simulink library "nmc"  (R2015b)
settings: Solver=ode45  SolverMode=SingleTasking  StartTime=0.0  StopTime=10.0  RelTol=1e-3
undefined symbols (not defined in the file): AFOFS_DIM, alphaFmGas, alphaFmGlu, alphaFmHam, alphaFmSol, alphaFmVas, alphaLceHam, alphaLceHfl, alphaLceTa, alphaLceTa1, Amp, amp_var, c, c_jointstop, CPG, D1G_HAT, DeltaThRef, eref, FmaxGAS, FmaxGLU, FmaxHAM, FmaxHFL, FmaxSOL, FmaxTA, FmaxVAS, freq, freq_var, GainDeltaTheta, GainGAS, GainGLU, GainHAM, GainHAMHFL, GainHFL, GainKneOverExt, GainSOL, GainSOLTA, GainTA, GainVAS, K, K_swing, KneePh23Offset, LceOffsetHAM, LceOffsetHFL, LceOffsetTA, left, LongDelay, loptGAS, loptGLU, loptHAM, loptHFL, loptSOL, loptTA, loptVAS, Lphi230, lslackGAS, lslackGLU, lslackHAM, lslackHFL, lslackSOL, lslackTA ... (+66)
libraries: nmc x94, simulink x29, simulink_extras x17
(part 2 of 5)

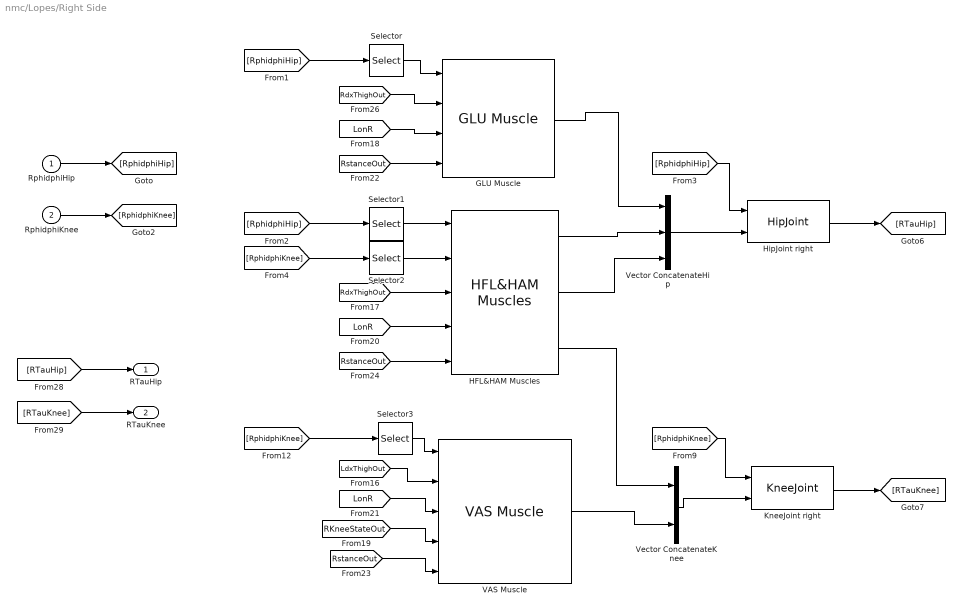
== system nmc/Lopes/Right Side ==
  RphidphiHip : Inport
  RphidphiKnee : Inport  Port=2
  GLU Muscle : nmc/NMC Muscles/GLU Muscle  StimGluSide=StimGLUR  GotoTag=GLUR_VM
  HFL&HAM Muscles : nmc/NMC Muscles/HFL&HAM Muscles  StimHAMSide=StimHAMR  StimHFLSide=StimHFLR  HAMVM=HAMR_VM  HFLVM=HFLR_VM
  HipJoint right : nmc/NMC Joints/HipJoint
  KneeJoint right : nmc/NMC Joints/KneeJoint
  Selector{,1..3} (4 alike) : Selector  InputPortWidth=2  IndexOptions=Index vector (dialog)  Indices=[1 ]  OutputSizes=1
  VAS Muscle : nmc/NMC Muscles/VAS Muscle  VariableName=StimVASR  VASVM=VASR_VM
  Vector ConcatenateHip : Concatenate  NumInputs=3
  Vector ConcatenateKnee : Concatenate
  RTauHip : Outport
  RTauKnee : Outport  Port=2
  wires:
  Vector ConcatenateHip/1 -> HipJoint right/2
  [RphidphiKnee] -> KneeJoint right/1
  Selector1/1 -> HFL&HAM Muscles/1
  [LdxThighOut] -> VAS Muscle/2
  Vector ConcatenateKnee/1 -> KneeJoint right/2
  Selector3/1 -> VAS Muscle/1
  VAS Muscle/1 -> Vector ConcatenateKnee/2
  HFL&HAM Muscles/1 -> Vector ConcatenateHip/2
  GLU Muscle/1 -> Vector ConcatenateHip/1
  [LonR] -> VAS Muscle/3
  [RphidphiKnee] -> Selector3/1
  [RKneeStateOut] -> VAS Muscle/4
  HFL&HAM Muscles/3 -> Vector ConcatenateKnee/1
  Selector/1 -> GLU Muscle/1
  HFL&HAM Muscles/2 -> Vector ConcatenateHip/3
  Selector2/1 -> HFL&HAM Muscles/2
  [RphidphiHip] -> Selector1/1
  [RstanceOut] -> VAS Muscle/5
  [RphidphiHip] -> Selector/1
  [RphidphiHip] -> HipJoint right/1
  [RphidphiKnee] -> Selector2/1
  HipJoint right/1 -> [RTauHip]
  KneeJoint right/1 -> [RTauKnee]
  [RdxThighOut] -> GLU Muscle/2
  [LonR] -> GLU Muscle/3
  [RstanceOut] -> GLU Muscle/4
  [RdxThighOut] -> HFL&HAM Muscles/3
  [LonR] -> HFL&HAM Muscles/4
  [RstanceOut] -> HFL&HAM Muscles/5
  RphidphiHip/1 -> [RphidphiHip]
  RphidphiKnee/1 -> [RphidphiKnee]
  [RTauHip] -> RTauHip/1
  [RTauKnee] -> RTauKnee/1

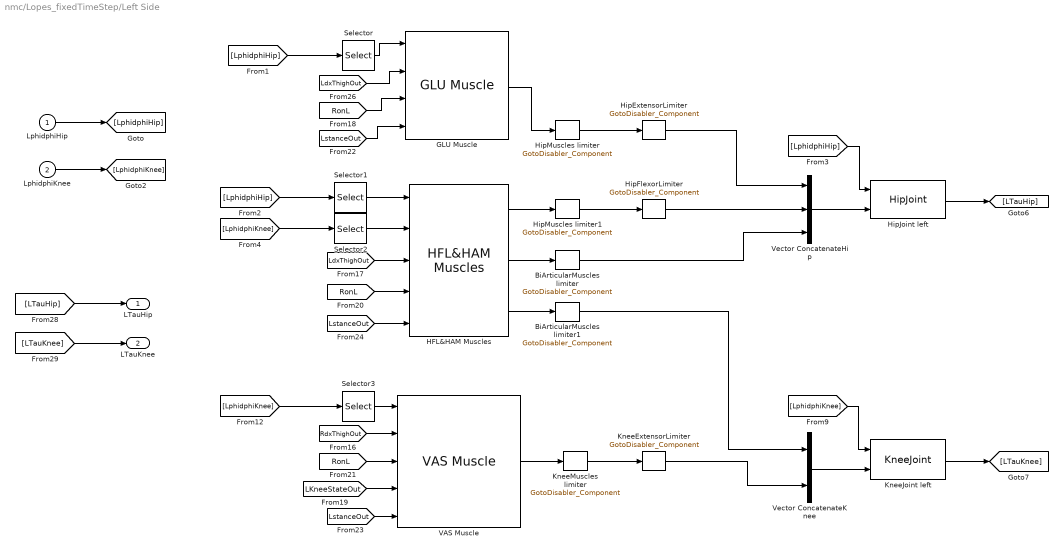
== system nmc/Lopes_fixedTimeStep/Left Side ==
  LphidphiHip : Inport
  LphidphiKnee : Inport  Port=2
  BiArticularMuscles limiter : nmc/GotoDisabler_Component  GotoTag=NMC_BiArticularMuscles_Percentage
  BiArticularMuscles limiter1 : nmc/GotoDisabler_Component  GotoTag=NMC_BiArticularMuscles_Percentage
  GLU Muscle : nmc/NMC Muscles/GLU Muscle  StimGluSide=StimGLUL  GotoTag=GLUR_VM
  HFL&HAM Muscles : nmc/NMC Muscles/HFL&HAM Muscles  StimHAMSide=StimHAML  StimHFLSide=StimHFLL  HAMVM=HAMR_VM  HFLVM=HFLR_VM
  HipExtensorLimiter : nmc/GotoDisabler_Component  GotoTag=NMC_HipExtensors_Percentage
  HipFlexorLimiter : nmc/GotoDisabler_Component  GotoTag=NMC_HipFlexors_Percentage
  HipJoint left : nmc/NMC Joints/HipJoint
  HipMuscles limiter : nmc/GotoDisabler_Component  GotoTag=NMC_HipMuscles_Percentage
  HipMuscles limiter1 : nmc/GotoDisabler_Component  GotoTag=NMC_HipMuscles_Percentage
  KneeExtensorLimiter : nmc/GotoDisabler_Component  GotoTag=NMC_KneeExtensors_Percentage
  KneeJoint left : nmc/NMC Joints/KneeJoint
  KneeMuscles limiter : nmc/GotoDisabler_Component  GotoTag=NMC_KneeMuscles_Percentage
  Selector{,1..3} (4 alike) : Selector  InputPortWidth=2  IndexOptions=Index vector (dialog)  Indices=[1 ]  OutputSizes=1
  VAS Muscle : nmc/NMC Muscles/VAS Muscle  VariableName=StimVASL  VASVM=VASR_VM
  Vector ConcatenateHip : Concatenate  NumInputs=3
  Vector ConcatenateKnee : Concatenate
  LTauHip : Outport
  LTauKnee : Outport  Port=2
  wires:
  KneeExtensorLimiter/1 -> Vector ConcatenateKnee/2
  BiArticularMuscles limiter1/1 -> Vector ConcatenateKnee/1
  HipFlexorLimiter/1 -> Vector ConcatenateHip/2
  HipExtensorLimiter/1 -> Vector ConcatenateHip/1
  KneeMuscles limiter/1 -> KneeExtensorLimiter/1
  BiArticularMuscles limiter/1 -> Vector ConcatenateHip/3
  HipMuscles limiter1/1 -> HipFlexorLimiter/1
  HipMuscles limiter/1 -> HipExtensorLimiter/1
  HFL&HAM Muscles/3 -> BiArticularMuscles limiter1/1
  GLU Muscle/1 -> HipMuscles limiter/1
  [LTauKnee] -> LTauKnee/1
  [LTauHip] -> LTauHip/1
  LphidphiKnee/1 -> [LphidphiKnee]
  LphidphiHip/1 -> [LphidphiHip]
  [LdxThighOut] -> HFL&HAM Muscles/3
  [RonL] -> GLU Muscle/3
  [LstanceOut] -> GLU Muscle/4
  [LdxThighOut] -> GLU Muscle/2
  KneeJoint left/1 -> [LTauKnee]
  HipJoint left/1 -> [LTauHip]
  [LphidphiKnee] -> Selector2/1
  [LphidphiHip] -> HipJoint left/1
  [LphidphiHip] -> Selector/1
  [LstanceOut] -> VAS Muscle/5
  [LphidphiHip] -> Selector1/1
  Selector2/1 -> HFL&HAM Muscles/2
  HFL&HAM Muscles/2 -> BiArticularMuscles limiter/1
  Selector/1 -> GLU Muscle/1
  [LKneeStateOut] -> VAS Muscle/4
  [RonL] -> HFL&HAM Muscles/4
  [LphidphiKnee] -> Selector3/1
  [RonL] -> VAS Muscle/3
  [LstanceOut] -> HFL&HAM Muscles/5
  HFL&HAM Muscles/1 -> HipMuscles limiter1/1
  VAS Muscle/1 -> KneeMuscles limiter/1
  Selector3/1 -> VAS Muscle/1
  Vector ConcatenateKnee/1 -> KneeJoint left/2
  [RdxThighOut] -> VAS Muscle/2
  Selector1/1 -> HFL&HAM Muscles/1
  [LphidphiKnee] -> KneeJoint left/1
  Vector ConcatenateHip/1 -> HipJoint left/2

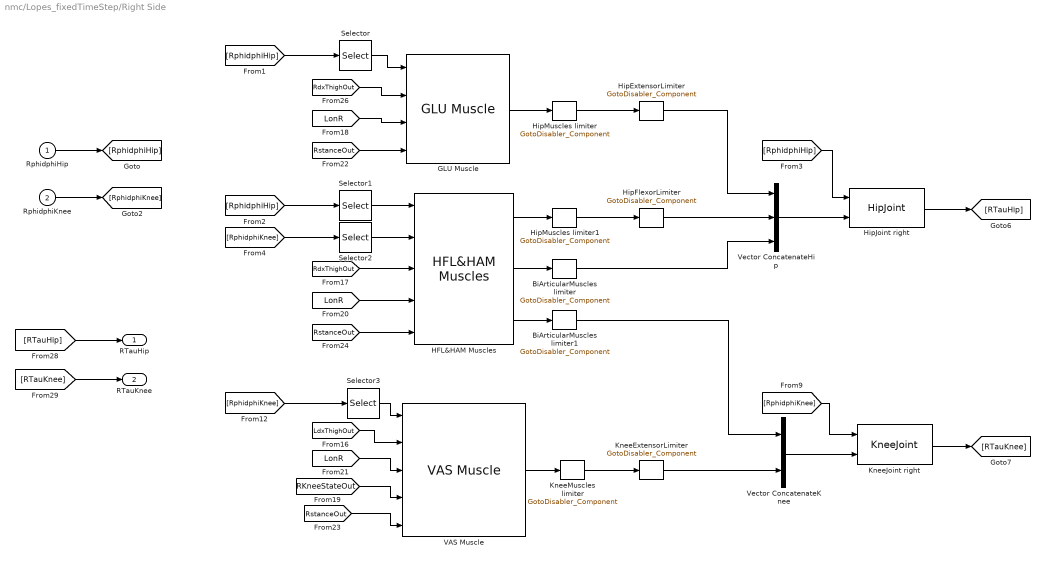
== system nmc/Lopes_fixedTimeStep/Right Side ==
  RphidphiHip : Inport
  RphidphiKnee : Inport  Port=2
  BiArticularMuscles limiter : nmc/GotoDisabler_Component  GotoTag=NMC_BiArticularMuscles_Percentage
  BiArticularMuscles limiter1 : nmc/GotoDisabler_Component  GotoTag=NMC_BiArticularMuscles_Percentage
  GLU Muscle : nmc/NMC Muscles/GLU Muscle  StimGluSide=StimGLUR  GotoTag=GLUR_VM
  HFL&HAM Muscles : nmc/NMC Muscles/HFL&HAM Muscles  StimHAMSide=StimHAMR  StimHFLSide=StimHFLR  HAMVM=HAMR_VM  HFLVM=HFLR_VM
  HipExtensorLimiter : nmc/GotoDisabler_Component  GotoTag=NMC_HipExtensors_Percentage
  HipFlexorLimiter : nmc/GotoDisabler_Component  GotoTag=NMC_HipFlexors_Percentage
  HipJoint right : nmc/NMC Joints/HipJoint
  HipMuscles limiter : nmc/GotoDisabler_Component  GotoTag=NMC_HipMuscles_Percentage
  HipMuscles limiter1 : nmc/GotoDisabler_Component  GotoTag=NMC_HipMuscles_Percentage
  KneeExtensorLimiter : nmc/GotoDisabler_Component  GotoTag=NMC_KneeExtensors_Percentage
  KneeJoint right : nmc/NMC Joints/KneeJoint
  KneeMuscles limiter : nmc/GotoDisabler_Component  GotoTag=NMC_KneeMuscles_Percentage
  Selector{,1..3} (4 alike) : Selector  InputPortWidth=2  IndexOptions=Index vector (dialog)  Indices=[1 ]  OutputSizes=1
  VAS Muscle : nmc/NMC Muscles/VAS Muscle  VariableName=StimVASR  VASVM=VASR_VM
  Vector ConcatenateHip : Concatenate  NumInputs=3
  Vector ConcatenateKnee : Concatenate
  RTauHip : Outport
  RTauKnee : Outport  Port=2
  wires:
  KneeExtensorLimiter/1 -> Vector ConcatenateKnee/2
  BiArticularMuscles limiter1/1 -> Vector ConcatenateKnee/1
  HipFlexorLimiter/1 -> Vector ConcatenateHip/2
  HipExtensorLimiter/1 -> Vector ConcatenateHip/1
  KneeMuscles limiter/1 -> KneeExtensorLimiter/1
  BiArticularMuscles limiter/1 -> Vector ConcatenateHip/3
  HipMuscles limiter1/1 -> HipFlexorLimiter/1
  HipMuscles limiter/1 -> HipExtensorLimiter/1
  [RTauKnee] -> RTauKnee/1
  [RTauHip] -> RTauHip/1
  RphidphiKnee/1 -> [RphidphiKnee]
  RphidphiHip/1 -> [RphidphiHip]
  [RstanceOut] -> HFL&HAM Muscles/5
  [LonR] -> HFL&HAM Muscles/4
  [RdxThighOut] -> HFL&HAM Muscles/3
  [RstanceOut] -> GLU Muscle/4
  [LonR] -> GLU Muscle/3
  [RdxThighOut] -> GLU Muscle/2
  KneeJoint right/1 -> [RTauKnee]
  HipJoint right/1 -> [RTauHip]
  [RphidphiKnee] -> Selector2/1
  [RphidphiHip] -> HipJoint right/1
  [RphidphiHip] -> Selector/1
  [RstanceOut] -> VAS Muscle/5
  [RphidphiHip] -> Selector1/1
  Selector2/1 -> HFL&HAM Muscles/2
  HFL&HAM Muscles/2 -> BiArticularMuscles limiter/1
  Selector/1 -> GLU Muscle/1
  HFL&HAM Muscles/3 -> BiArticularMuscles limiter1/1
  [RKneeStateOut] -> VAS Muscle/4
  [RphidphiKnee] -> Selector3/1
  [LonR] -> VAS Muscle/3
  GLU Muscle/1 -> HipMuscles limiter/1
  HFL&HAM Muscles/1 -> HipMuscles limiter1/1
  VAS Muscle/1 -> KneeMuscles limiter/1
  Selector3/1 -> VAS Muscle/1
  Vector ConcatenateKnee/1 -> KneeJoint right/2
  [LdxThighOut] -> VAS Muscle/2
  Selector1/1 -> HFL&HAM Muscles/1
  [RphidphiKnee] -> KneeJoint right/1
  Vector ConcatenateHip/1 -> HipJoint right/2

== system nmc/NMC Joints/AnkleJoint ==
  note: Ankle Joint
  phidphiAnkle : Inport
  PreTauAnkle : Inport  Port=2
  " Ankle Joint Limits" : Subsystem
  Demux : Demux  Outputs=2
  GotoDisabler_Component : nmc/GotoDisabler_Component  GotoTag=EnableNMC_JointLimits
  LOG_TauAnkleLigament : Concatenate  NumInputs=1
  Sum : Sum  Inputs=|++
  Sum of Elements : Sum  Inputs=+
  TauAnkle : Outport
  wires:
  Demux/1 -> " Ankle Joint Limits"/1(phi [rad])
  Demux/2 -> " Ankle Joint Limits"/2(dphi [rad/s])
  PreTauAnkle/1 -> Sum of Elements/1
  phidphiAnkle/1 -> Demux/1
  " Ankle Joint Limits"/1(M_stop [Nm]) -> LOG_TauAnkleLigament/1
  Sum/1 -> TauAnkle/1
  Sum of Elements/1 -> Sum/2
  LOG_TauAnkleLigament/1 -> GotoDisabler_Component/1
  GotoDisabler_Component/1 -> Sum/1

== system nmc/NMC Joints/HipJoint ==
  note: Hip Joint
  phidphiHip : Inport
  PreTauHip : Inport  Port=2
  Demux2 : Demux  Outputs=2
  GotoDisabler_Component : nmc/GotoDisabler_Component  GotoTag=DisableNMC_JointLimits
  Hip Joint Limits : Subsystem
  Sum of Elements : Sum  Inputs=+
  Sum16 : Sum  Inputs=|++
  TauHip : Outport
  wires:
  phidphiHip/1 -> Demux2/1
  Demux2/1 -> Hip Joint Limits/1(phi [rad])
  Demux2/2 -> Hip Joint Limits/2(dphi [rad/s])
  Hip Joint Limits/1(M_stop [Nm]) -> GotoDisabler_Component/1
  Sum16/1 -> TauHip/1
  PreTauHip/1 -> Sum of Elements/1
  Sum of Elements/1 -> Sum16/2
  GotoDisabler_Component/1 -> Sum16/1

== system nmc/NMC Joints/KneeJoint ==
  note: Knee Joint
  phidphiKnee : Inport
  PreTauKnee : Inport  Port=2
  Demux1 : Demux  Outputs=2
  Gain : Gain  Gain=-1
  GotoDisabler_Component : nmc/GotoDisabler_Component  GotoTag=DisableNMC_JointLimits
  Knee Joint Limits : Subsystem
  Sum : Sum  Inputs=|++
  Sum of Elements : Sum  Inputs=+
  TauKnee : Outport
  wires:
  Demux1/1 -> Knee Joint Limits/1(phi [rad])
  Demux1/2 -> Knee Joint Limits/2(dphi [rad/s])
  phidphiKnee/1 -> Demux1/1
  Knee Joint Limits/1(M_stop [Nm]) -> GotoDisabler_Component/1
  Sum/1 -> TauKnee/1
  PreTauKnee/1 -> Sum of Elements/1
  Sum of Elements/1 -> Gain/1
  Gain/1 -> Sum/2
  GotoDisabler_Component/1 -> Sum/1

== system nmc/NMC Muscles/GAS Muscle ==
  note: GAS Muscle
  phiKnee : Inport
  phiAnkle : Inport  Port=2
  StanceSwing : Inport  Port=3
  "GAS Actuation " : Subsystem
  GAS Control : Subsystem
  LOG_GasAnkle : Concatenate  NumInputs=1
  LOG_TauGasKnee : Concatenate  NumInputs=1
  StimGAS : ToWorkspace  VariableName=StimGAS  SaveFormat=Timeseries  SampleTime=-1
  TauGasKnee : Outport
  TauGasAnkle : Outport  Port=2
  wires:
  GAS Control/1(StimGAS) -> "GAS Actuation "/3(StimGas), StimGAS/1
  phiKnee/1 -> "GAS Actuation "/1(phiKnee)
  StanceSwing/1 -> GAS Control/2(StanceSwing)
  "GAS Actuation "/3(FmGas) -> GAS Control/1(FmGAS)
  "GAS Actuation "/2(TauGasAnkle) -> LOG_GasAnkle/1
  "GAS Actuation "/1(TauGasKnee) -> LOG_TauGasKnee/1
  phiAnkle/1 -> "GAS Actuation "/2(phiAnkle)
  LOG_TauGasKnee/1 -> TauGasKnee/1
  LOG_GasAnkle/1 -> TauGasAnkle/1

== system nmc/NMC Muscles/GLU Muscle ==
  note: GLU Muscle
  phiHip : Inport
  CLdxThigh : Inport  Port=2
  OLonCL : Inport  Port=3
  StanceSwing : Inport  Port=4
  GLU Actuation : Subsystem
  GLU Control : Subsystem
  LOG_TauGlu : Concatenate  NumInputs=1
  StimGLU : ToWorkspace  VariableName=StimGLUR  SaveFormat=Timeseries  SampleTime=-1
  TauGlu : Outport
  wires:
  GLU Actuation/1(TauGlu) -> LOG_TauGlu/1
  StanceSwing/1 -> GLU Control/6(StanceSwing)
  CLdxThigh/1 -> GLU Control/4(CLdxThigh)
  phiHip/1 -> GLU Actuation/1(phiHip)
  [dThetaDelayed] -> GLU Control/3(dTheta)
  [ThetaDelayed] -> GLU Control/2(Theta)
  OLonCL/1 -> GLU Control/5(OLonCL)
  GLU Actuation/2(FmGlu) -> GLU Control/1(FmGlu)
  GLU Control/1(StimGlu) -> StimGLU/1, GLU Actuation/2(StimGlu)
  LOG_TauGlu/1 -> TauGlu/1

== system nmc/NMC Muscles/HFL Muscle  ==
  note: HFL Muscle
  phiHip : Inport
  CLdxThigh : Inport  Port=2
  OLonCL : Inport  Port=3
  StanceSwing : Inport  Port=4
  HFL Actuation : Subsystem
  HFL Control : Subsystem
  LOG_TauHFL : Concatenate  NumInputs=1
  StimHFL : ToWorkspace  VariableName=StimHFL  SaveFormat=Timeseries  SampleTime=-1
  TauHFL : Outport
  wires:
  HFL Actuation/1(TauHFL) -> LOG_TauHFL/1
  phiHip/1 -> HFL Actuation/1(phiHip)
  StanceSwing/1 -> HFL Control/6(StanceSwing)
  OLonCL/1 -> HFL Control/5(OLonCL)
  CLdxThigh/1 -> HFL Control/4(CLdxThigh)
  [dThetaDelayed] -> HFL Control/3(dTheta)
  [ThetaDelayed] -> HFL Control/2(Theta)
  HFL Control/1(StimHFL) -> HFL Actuation/2(StimHFL), StimHFL/1
  HFL Actuation/2(LceHFL) -> HFL Control/1(LceHFL)
  LOG_TauHFL/1 -> TauHFL/1

== system nmc/NMC Muscles/HFL&HAM Muscles ==
  note: HFL&HAM Muscles
  phiHip : Inport
  phiKnee : Inport  Port=2
  CLdxThigh : Inport  Port=3
  OLonCL : Inport  Port=4
  StanceSwing : Inport  Port=5
  "HAM Actuation " : Subsystem
  HFL Actuation : Subsystem
  HFL&HAM Control : Subsystem
  LOG_TauHFL : Concatenate  NumInputs=1
  LOG_TauHamHip : Concatenate  NumInputs=1
  LOG_TauHamKnee : Concatenate  NumInputs=1
  StimHAM : ToWorkspace  VariableName=StimHAMR  SaveFormat=Timeseries  SampleTime=-1
  StimHFL : ToWorkspace  VariableName=StimHFLR  SaveFormat=Timeseries  SampleTime=-1
  TauHFL : Outport
  TauHamHip : Outport  Port=2
  TauHamKnee : Outport  Port=3
  wires:
  HFL&HAM Control/1(StimHFL) -> HFL Actuation/2(StimHFL), StimHFL/1
  "HAM Actuation "/3(LceHam) -> HFL&HAM Control/2(LceHam)
  "HAM Actuation "/4(FmHam) -> HFL&HAM Control/3(FmHam)
  HFL Actuation/2(LceHFL) -> HFL&HAM Control/1(LceHFL)
  OLonCL/1 -> HFL&HAM Control/7(OLonCL)
  "HAM Actuation "/1(TauHamHip) -> LOG_TauHamHip/1
  phiHip/1 -> HFL Actuation/1(phiHip), "HAM Actuation "/1(phiHip)
  "HAM Actuation "/2(TauHamKnee) -> LOG_TauHamKnee/1
  CLdxThigh/1 -> HFL&HAM Control/6(CLdxThigh)
  HFL Actuation/1(TauHFL) -> LOG_TauHFL/1
  phiKnee/1 -> "HAM Actuation "/2(phiKnee)
  [ThetaDelayed] -> HFL&HAM Control/4(Theta)
  [dThetaDelayed] -> HFL&HAM Control/5(dTheta)
  StanceSwing/1 -> HFL&HAM Control/8(StanceSwing)
  HFL&HAM Control/2(StimHAM) -> "HAM Actuation "/3(StimHam), StimHAM/1
  LOG_TauHFL/1 -> TauHFL/1
  LOG_TauHamHip/1 -> TauHamHip/1
  LOG_TauHamKnee/1 -> TauHamKnee/1

== system nmc/NMC Muscles/SOL&TA Muscles ==
  note: SOL&TA Muscles
  phiAnkle : Inport
  StanceSwing : Inport  Port=2
  LOG_StimSOL : Concatenate  NumInputs=1
  LOG_StimTA : Concatenate  NumInputs=1
  LOG_TauSOL : Concatenate  NumInputs=1
  LOG_TauTA : Concatenate  NumInputs=1
  SOL Actuation : Subsystem
  SOL&TA Control : Subsystem
  StimSOL : ToWorkspace  VariableName=StimSOL  SaveFormat=Timeseries  SampleTime=-1
  StimTA : ToWorkspace  VariableName=StimTA  SaveFormat=Timeseries  SampleTime=-1
  TA Actuation : Subsystem
  TauTA : Outport
  TauSOL : Outport  Port=2
  wires:
  SOL&TA Control/2(StimSOL) -> LOG_StimSOL/1
  SOL Actuation/2(FmSOL) -> SOL&TA Control/2(FmSOL)
  SOL Actuation/1(TauSOL) -> LOG_TauSOL/1
  SOL&TA Control/1(StimTA) -> LOG_StimTA/1
  StanceSwing/1 -> SOL&TA Control/3(StanceSwing)
  TA Actuation/1(LceTA) -> SOL&TA Control/1(LceTA)
  phiAnkle/1 -> TA Actuation/1(phiAnkle), SOL Actuation/1(phiAnkle)
  TA Actuation/2(TauTa) -> LOG_TauTA/1
  LOG_TauTA/1 -> TauTA/1
  LOG_TauSOL/1 -> TauSOL/1
  LOG_StimTA/1 -> StimTA/1, TA Actuation/2(StimTA)
  LOG_StimSOL/1 -> SOL Actuation/2(StimSOL), StimSOL/1

== system nmc/NMC Muscles/VAS Muscle ==
  note: VAS Muscle
  phiKnee : Inport
  OLdxThigh : Inport  Port=2
  OLonCL : Inport  Port=3
  CLKneeState : Inport  Port=4
  StanceSwing : Inport  Port=5
  LOG_TauVas : Concatenate  NumInputs=1
  StimVAS : ToWorkspace  VariableName=StimVASR  SaveFormat=Timeseries  SampleTime=-1
  "VAS Actuation " : Subsystem
  VAS Control : Subsystem
  TauVas : Outport
  wires:
  CLKneeState/1 -> VAS Control/4(CLKneeState)
  phiKnee/1 -> "VAS Actuation "/1(phiKnee)
  OLdxThigh/1 -> VAS Control/2(OLdxThigh)
  StanceSwing/1 -> VAS Control/5(StanceSwing)
  OLonCL/1 -> VAS Control/3(OLonCL)
  "VAS Actuation "/1(TauVas) -> LOG_TauVas/1
  "VAS Actuation "/2(FmVas) -> VAS Control/1(FmVAS)
  VAS Control/1(StimVAS) -> "VAS Actuation "/2(StimVas), StimVAS/1
  LOG_TauVas/1 -> TauVas/1

== system nmc/NMC Sensors/FootSensor ==
  note: Muscle
      | Actuation
      | Layer
      | Interface
      | (Right
      | Muscle
      | Sensors)
  note: Muscle
      | Actuation
      | Layer
      | Interface
      | (Left
      | Muscle
      | Sensors)
  note: Body Mechanics Layer Interface
      | (Foot Skin Sensors)
  LStance : Inport
  RStance : Inport  Port=2
  Cross Influence Detection : Subsystem
  Cross Influence Detection1 : Subsystem  Commented=on
  Data Type Conversion : DataTypeConversion
  Data Type Conversion1 : DataTypeConversion
  L Stance afferent delay : TransportDelay  DelayTime=MidDelay
  L_switch_signal : nmc/L_switch_signal
  R Stance afferent delay : TransportDelay  DelayTime=MidDelay
  R_switch_signal : nmc/R_switch_signal
  Terminator : Terminator
  To Workspace : ToWorkspace  VariableName=Stance  SaveFormat=Timeseries  SampleTime=-1
  To Workspace1 : ToWorkspace  VariableName=RonLLonR  SaveFormat=Timeseries  SampleTime=-1
  Vector ConcatenateHip : Concatenate
  Vector ConcatenateHip1 : Concatenate
  LStanceOut : Outport
  RstanceOut : Outport  Port=2
  LonR : Outport  Port=3
  RonL : Outport  Port=4
  wires:
  Data Type Conversion1/1 -> R Stance afferent delay/1
  Data Type Conversion/1 -> L Stance afferent delay/1
  Vector ConcatenateHip/1 -> To Workspace1/1
  Cross Influence Detection/3(LonR) -> LonR/1, Vector ConcatenateHip/2
  Cross Influence Detection/1(RonL) -> RonL/1, Vector ConcatenateHip/1
  Vector ConcatenateHip1/1 -> To Workspace/1
  R Stance afferent delay/1 -> RstanceOut/1, Vector ConcatenateHip1/2, R_switch_signal/1, Cross Influence Detection/2(RStance)
  L Stance afferent delay/1 -> LStanceOut/1, L_switch_signal/1, Vector ConcatenateHip1/1, Cross Influence Detection/1(LStance)
  RStance/1 -> Data Type Conversion1/1
  LStance/1 -> Data Type Conversion/1
  Cross Influence Detection/2(Flight) -> Terminator/1

== system nmc/NMC Sensors/FootSensorSimple ==
  note: Body Mechanics Layer Interface
      | (Foot Skin Sensors)
  LStance : Inport
  RStance : Inport  Port=2
  L Stance afferent delay : TransportDelay  DelayTime=MidDelay
  R Stance afferent delay : TransportDelay  DelayTime=MidDelay
  LstanceOut : Outport
  RstanceOut : Outport  Port=2
  wires:
  LStance/1 -> L Stance afferent delay/1
  RStance/1 -> R Stance afferent delay/1
  L Stance afferent delay/1 -> LstanceOut/1
  R Stance afferent delay/1 -> RstanceOut/1

== system nmc/NMC Sensors/FootSensor_fixedTimestep ==
  note: Body Mechanics Layer Interface
      | (Foot Skin Sensors)
  LStance : Inport
  RStance : Inport  Port=2
  Cross Influence Detection_fixedTimestep : nmc/Cross Influence Detection_fixedTimestep
  Data Type Conversion : DataTypeConversion
  Data Type Conversion1 : DataTypeConversion
  L Stance afferent delay : TransportDelay  DelayTime=MidDelay
  L_switch_signal : nmc/L_switch_signal
  R Stance afferent delay : TransportDelay  DelayTime=MidDelay
  R_switch_signal : nmc/R_switch_signal
  Switch : Switch  Criteria=u2 > Threshold
  Switch2 : Switch  Criteria=u2 > Threshold
  Terminator : Terminator
  To Workspace : ToWorkspace  VariableName=Stance  SaveFormat=Timeseries  SampleTime=-1
  To Workspace1 : ToWorkspace  VariableName=RonLLonR  SaveFormat=Timeseries  SampleTime=-1
  Vector ConcatenateHip : Concatenate
  Vector ConcatenateHip1 : Concatenate
  LStanceOut : Outport
  RstanceOut : Outport  Port=2
  LonR : Outport  Port=3
  RonL : Outport  Port=4
  wires:
  Switch2/1 -> RstanceOut/1, Cross Influence Detection_fixedTimestep/2
  Switch/1 -> Cross Influence Detection_fixedTimestep/1, LStanceOut/1
  R Stance afferent delay/1 -> Switch2/1
  L Stance afferent delay/1 -> Switch/1
  [EnableGaitPhaseDelay] -> Switch2/2, Switch/2
  Cross Influence Detection_fixedTimestep/2 -> Terminator/1
  LStance/1 -> Data Type Conversion/1
  RStance/1 -> Data Type Conversion1/1
  Vector ConcatenateHip1/1 -> To Workspace/1
  Cross Influence Detection_fixedTimestep/1 -> Vector ConcatenateHip/1, RonL/1
  Cross Influence Detection_fixedTimestep/3 -> Vector ConcatenateHip/2, LonR/1
  Vector ConcatenateHip/1 -> To Workspace1/1
  Data Type Conversion/1 -> L Stance afferent delay/1, Switch/3
  Data Type Conversion1/1 -> R Stance afferent delay/1, Switch2/3

== system nmc/NMC Sensors/GeyerUpperBodyOrientation ==
  note: Upper Body Orientation
  xyzLHip : Inport
  xyzRHip : Inport  Port=2
  dxyzLHip : Inport  Port=3
  dxyzRHip : Inport  Port=4
  xyzHAT : Inport  Port=5
  dxyzHAT : Inport  Port=6
  " Mean Hip Speed" : Gain  Gain=1/2
  "Dx, Dy" : Selector  InputPortWidth=3  IndexOptions=Index vector (dialog)  Indices=[1 2]  OutputSizes=1
  Mean Hip Position : Gain  Gain=1/2
  Mux2 : Mux  Inputs=2
  Sum1 : Sum
  Sum2 : Sum
  Sum4 : Sum  Inputs=-+
  Sum5 : Sum  Inputs=+-
  To Workspace : ToWorkspace  VariableName=xHipdxHip  SaveFormat=Timeseries  SampleTime=-1
  To Workspace2 : ToWorkspace  VariableName=xHatdxHat  SaveFormat=Timeseries  SampleTime=-1
  Vector ConcatenateHip : Concatenate
  Vector ConcatenateHip2 : Concatenate
  dDx : Selector  InputPortWidth=3  IndexOptions=Index vector (dialog)  Indices=[1 2]  OutputSizes=1
  dtheta : Fcn  Expr=( u(2)*u(3) - u(1)*u(4) ) / D1G_HAT^2
  theta : Fcn  Expr=atan2(u(1),u(2))
  Theta : Outport
  dTheta : Outport  Port=2
  wires:
  Vector ConcatenateHip/1 -> To Workspace2/1
  Vector ConcatenateHip2/1 -> To Workspace/1
  Sum4/1 -> "Dx, Dy"/1
  dxyzHAT/1 -> Sum5/1, Vector ConcatenateHip/2
  Sum5/1 -> dDx/1
  dDx/1 -> Mux2/2
  Mux2/1 -> dtheta/1
  xyzLHip/1 -> Sum1/1
  Sum1/1 -> Mean Hip Position/1
  Sum2/1 -> " Mean Hip Speed"/1
  Mean Hip Position/1 -> Sum4/1, Vector ConcatenateHip2/1
  " Mean Hip Speed"/1 -> Sum5/2, Vector ConcatenateHip2/2
  theta/1 -> Theta/1
  dtheta/1 -> dTheta/1
  "Dx, Dy"/1 -> Mux2/1, theta/1
  xyzRHip/1 -> Sum1/2
  dxyzLHip/1 -> Sum2/1
  xyzHAT/1 -> Sum4/2, Vector ConcatenateHip/1
  dxyzRHip/1 -> Sum2/2

== system nmc/NMC Sensors/KneeSensor ==
  note: Body Mechanics Layer Interface
      | (Knee Sensors)
  LKneeState : Inport
  RKneeState : Inport  Port=2
  Demux1 : Demux  Outputs=2
  Demux2 : Demux  Outputs=2
  L Knee loop delay : TransportDelay  DelayTime=MidDelay
  Mux1 : Mux  Inputs=2
  Mux6 : Mux  Inputs=2
  R Knee loop delay : TransportDelay  DelayTime=MidDelay
  Stimulation Bias1 : Constant  Value=KneePh23Offset
  Stimulation Bias10 : Constant  Value=KneePh23Offset
  Sum1 : Sum  Inputs=-+|  SaturateOnIntegerOverflow=on  InputSameDT=on  OutDataTypeStr=Inherit: Same as first input
  Sum6 : Sum  Inputs=-+|  SaturateOnIntegerOverflow=on  InputSameDT=on  OutDataTypeStr=Inherit: Same as first input
  To Workspace : ToWorkspace  VariableName=KneeState  SaveFormat=Timeseries  SampleTime=-1
  Vector ConcatenateHip : Concatenate
  map (-pi,pi] to [0,2pi)1 : Fcn  Expr=u(1)*(u(1)>0)*(u(2)>0)
  map (-pi,pi] to [0,2pi)2 : Fcn  Expr=u(1)*(u(1)>0)*(u(2)>0)
  LKneeStateOut : Outport
  RKneeStateOut : Outport  Port=2
  wires:
  Vector ConcatenateHip/1 -> To Workspace/1
  RKneeState/1 -> Demux2/1
  Demux2/1 -> Sum6/2
  Demux2/2 -> Mux6/2
  Sum6/1 -> Mux6/1
  Mux6/1 -> map (-pi,pi] to [0,2pi)1/1
  map (-pi,pi] to [0,2pi)1/1 -> R Knee loop delay/1
  Stimulation Bias10/1 -> Sum6/1
  R Knee loop delay/1 -> RKneeStateOut/1, Vector ConcatenateHip/2
  LKneeState/1 -> Demux1/1
  Demux1/1 -> Sum1/2
  Demux1/2 -> Mux1/2
  Sum1/1 -> Mux1/1
  Mux1/1 -> map (-pi,pi] to [0,2pi)2/1
  map (-pi,pi] to [0,2pi)2/1 -> L Knee loop delay/1
  Stimulation Bias1/1 -> Sum1/1
  L Knee loop delay/1 -> LKneeStateOut/1, Vector ConcatenateHip/1

== system nmc/NMC Sensors/ThightSensor ==
  note: Body Mechanics Layer Interface
      | (Thigh Body Load Sensors)
  LdxThigh : Inport
  RdxThigh : Inport  Port=2
  L Thigh afferent delay : TransportDelay  DelayTime=ShortDelay
  R Thigh afferent delay : TransportDelay  DelayTime=ShortDelay
  To Workspace : ToWorkspace  VariableName=dxThight  SaveFormat=Timeseries  SampleTime=-1
  Vector ConcatenateHip : Concatenate
  smooth : TransferFcn  Denominator=[0.02 1]
  smooth1 : TransferFcn  Denominator=[0.02 1]
  LdxThighOut : Outport
  RdxThighOut : Outport  Port=2
  wires:
  Vector ConcatenateHip/1 -> To Workspace/1
  R Thigh afferent delay/1 -> RdxThighOut/1, Vector ConcatenateHip/2
  L Thigh afferent delay/1 -> LdxThighOut/1, Vector ConcatenateHip/1
  smooth1/1 -> R Thigh afferent delay/1
  LdxThigh/1 -> smooth/1
  smooth/1 -> L Thigh afferent delay/1
  RdxThigh/1 -> smooth1/1

== system nmc/NMC Sensors/ThightSensorSimulator ==
  note: Body Mechanics Layer Interface
      | (Thigh Body Load Sensors)
  LStance : Inport
  RStance : Inport  Port=2
  L Thigh afferent delay : TransportDelay  DelayTime=ShortDelay
  Maximum loading : Constant  Value=0.0069
  Product : Product
  Product1 : Product
  R Thigh afferent delay : TransportDelay  DelayTime=ShortDelay
  To Workspace : ToWorkspace  VariableName=dxThightNew  SaveFormat=Timeseries  SampleTime=-1
  Vector ConcatenateHip : Concatenate
  smooth : TransferFcn  Denominator=[0.02 1]
  smooth1 : TransferFcn  Denominator=[0.02 1]
  LdxThighOut : Outport
  RdxThighOut : Outport  Port=2
  wires:
  smooth/1 -> L Thigh afferent delay/1
  LStance/1 -> Product/2
  smooth1/1 -> R Thigh afferent delay/1
  L Thigh afferent delay/1 -> Vector ConcatenateHip/1, LdxThighOut/1
  R Thigh afferent delay/1 -> Vector ConcatenateHip/2, RdxThighOut/1
  Vector ConcatenateHip/1 -> To Workspace/1
  Product/1 -> smooth/1
  RStance/1 -> Product1/1
  Product1/1 -> smooth1/1
  Maximum loading/1 -> Product1/2, Product/1

== system nmc/NMC Sensors/UpperBodyOrientation ==
  note: Upper Body Orientation
  Theta : Inport
  dTheta : Inport  Port=2
  Body Pitch loop delay : TransportDelay  DelayTime=ShortDelay
  Body Pitch loop delay. : TransportDelay  DelayTime=ShortDelay
  tag scope: ThetaDelayed=global, dThetaDelayed=global
  wires:
  Theta/1 -> Body Pitch loop delay/1
  dTheta/1 -> Body Pitch loop delay./1
  Body Pitch loop delay/1 -> [ThetaDelayed]
  Body Pitch loop delay./1 -> [dThetaDelayed]

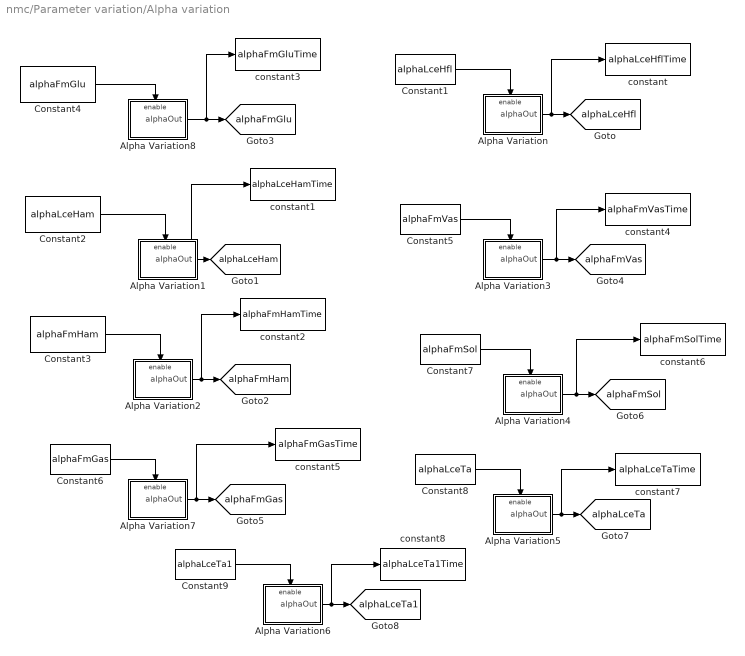
== system nmc/Parameter variation/Alpha variation ==
  Alpha Variation : Subsystem
  Alpha Variation1 : Subsystem
  Alpha Variation2 : Subsystem
  Alpha Variation3 : Subsystem
  Alpha Variation4 : Subsystem
  Alpha Variation5 : Subsystem
  Alpha Variation6 : Subsystem
  Alpha Variation7 : Subsystem
  Alpha Variation8 : Subsystem
  Constant1 : Constant  Value=alphaLceHfl
  Constant2 : Constant  Value=alphaLceHam
  Constant3 : Constant  Value=alphaFmHam
  Constant4 : Constant  Value=alphaFmGlu
  Constant5 : Constant  Value=alphaFmVas
  Constant6 : Constant  Value=alphaFmGas
  Constant7 : Constant  Value=alphaFmSol
  Constant8 : Constant  Value=alphaLceTa
  Constant9 : Constant  Value=alphaLceTa1
  constant : ToWorkspace  VariableName=alphaLceHflTime  SaveFormat=Timeseries  SampleTime=-1
  constant1 : ToWorkspace  VariableName=alphaLceHamTime  SaveFormat=Timeseries  SampleTime=-1
  constant2 : ToWorkspace  VariableName=alphaFmHamTime  SaveFormat=Timeseries  SampleTime=-1
  constant3 : ToWorkspace  VariableName=alphaFmGluTime  SaveFormat=Timeseries  SampleTime=-1
  constant4 : ToWorkspace  VariableName=alphaFmVasTime  SaveFormat=Timeseries  SampleTime=-1
  constant5 : ToWorkspace  VariableName=alphaFmGasTime  SaveFormat=Timeseries  SampleTime=-1
  constant6 : ToWorkspace  VariableName=alphaFmSolTime  SaveFormat=Timeseries  SampleTime=-1
  constant7 : ToWorkspace  VariableName=alphaLceTaTime  SaveFormat=Timeseries  SampleTime=-1
  constant8 : ToWorkspace  VariableName=alphaLceTa1Time  SaveFormat=Timeseries  SampleTime=-1
  tag scope: alphaFmGas=global, alphaFmGlu=global, alphaFmHam=global, alphaFmSol=global, alphaFmVas=global, alphaLceHam=global, alphaLceHfl=global, alphaLceTa1=global, alphaLceTa=global
  wires:
  Alpha Variation/1("alphaOut ") -> constant/1, [alphaLceHfl]
  Alpha Variation1/1("alphaOut ") -> constant1/1, [alphaLceHam]
  Alpha Variation2/1("alphaOut ") -> [alphaFmHam], constant2/1
  Constant3/1 -> Alpha Variation2/Enable
  Constant4/1 -> Alpha Variation8/Enable
  Alpha Variation8/1("alphaOut ") -> constant3/1, [alphaFmGlu]
  Constant5/1 -> Alpha Variation3/Enable
  Alpha Variation6/1("alphaOut ") -> constant8/1, [alphaLceTa1]
  Alpha Variation3/1("alphaOut ") -> constant4/1, [alphaFmVas]
  Alpha Variation7/1("alphaOut ") -> constant5/1, [alphaFmGas]
  Constant6/1 -> Alpha Variation7/Enable
  Constant7/1 -> Alpha Variation4/Enable
  Alpha Variation4/1("alphaOut ") -> constant6/1, [alphaFmSol]
  Alpha Variation5/1("alphaOut ") -> constant7/1, [alphaLceTa]
  Constant8/1 -> Alpha Variation5/Enable
  Constant9/1 -> Alpha Variation6/Enable
  Constant2/1 -> Alpha Variation1/Enable
  Constant1/1 -> Alpha Variation/Enable

== system nmc/Parameter variation/Amplitude Variation ==
  Add : Sum  Inputs=+++
  Constant1 : Constant  Value=amp_var
  Constant17 : Constant  Value=Amp
  Demux : Demux  Outputs=3
  Down : Subsystem
  "Off " : Subsystem
  Up : Subsystem
  constant10 : ToWorkspace  VariableName=ampTime  SaveFormat=Timeseries  SampleTime=-1
  tag scope: amp=global
  wires:
  Down/1("AmpDown ") -> Add/3
  Add/1 -> constant10/1, [amp]
  Demux/2 -> Up/Enable
  Demux/1 -> "Off "/Enable
  "Off "/1("Amp ") -> Add/1
  Constant1/1 -> Demux/1
  Demux/3 -> Down/Enable
  Up/1("AmpUp ") -> Add/2
  Constant17/1 -> Down/1(Amp), "Off "/1(Amp), Up/1(Amp)

== system nmc/Parameter variation/Freq variation ==
  Add : Sum  Inputs=+++
  Constant1 : Constant  Value=freq_var
  Constant17 : Constant  Value=freq
  Demux : Demux  Outputs=3
  Down : Subsystem
  "Off " : Subsystem
  Up : Subsystem
  constant10 : ToWorkspace  VariableName=freqTime  SaveFormat=Timeseries  SampleTime=-1
  tag scope: freq=global
  wires:
  Down/1("freqDown ") -> Add/3
  Add/1 -> constant10/1, [freq]
  Demux/2 -> Up/Enable
  Demux/1 -> "Off "/Enable
  "Off "/1("Amp ") -> Add/1
  Constant1/1 -> Demux/1
  Demux/3 -> Down/Enable
  Up/1("freqUp ") -> Add/2
  Constant17/1 -> Down/1("freq "), "Off "/1(freq), Up/1("freq ")

== system nmc/SynchonizedMorphOscillator/ConstantCPG ==
  cpg_cnst_value : Inport
  Enable : EnablePort
  cpg_value : Outport
  wires:
  cpg_cnst_value/1 -> cpg_value/1

== system nmc/SynchonizedMorphOscillator/MorphingOscillator ==
  g : Inport
  freq : Inport  Port=2
  switchsignal : Inport  Port=3
  swingOrstance : Inport  Port=4
  Derivative : Derivative
  K : Constant  Value=0
  Product : Product
  Product1 : Product
  Product2 : Product
  Subtract : Sum  Inputs=+-
  Sum : Sum  Inputs=|++
  Sum1 : Sum  Inputs=|++
  g_initial_condition : MATLAB Function  TreatAsAtomicUnit=on
  gamma : Gain  Gain=100
  modDg : MATLAB Function  TreatAsAtomicUnit=on
  "modg " : MATLAB Function  TreatAsAtomicUnit=on
  tetha : Integrator  ExternalReset=falling
  x : Integrator  ExternalReset=falling  InitialConditionSource=external
  cpg : Outport
  tetha_out : Outport  Port=2  InitialOutput=0
  wires:
  Product2/1 -> cpg/1
  Derivative/1 -> modDg/1(g)
  Sum1/1 -> x/1
  K/1 -> Sum1/2
  x/1 -> Subtract/2, Product2/1
  gamma/1 -> Sum/1
  "modg "/1(y) -> Subtract/1
  tetha/1 -> modDg/2(tetha), "modg "/2(tetha), tetha_out/1
  g/1 -> Derivative/1, g_initial_condition/1(g), "modg "/1(g)
  Subtract/1 -> gamma/1
  freq/1 -> Product/2, tetha/1
  modDg/1(y) -> Product/1
  Product/1 -> Sum/2
  Sum/1 -> Sum1/1
  switchsignal/1 -> Product1/1
  swingOrstance/1 -> Product1/2
  Product1/1 -> x/2, tetha/2
  g_initial_condition/1(y) -> x/3
  [amp] -> Product2/2

== system nmc/SynchonizedMorphOscillator/enable cpg ==
  cpg_on : Inport
  Enable : EnablePort
  cpg : Outport
  wires:
  cpg_on/1 -> cpg/1

== system nmc/VAS Muscle/VAS Actuation  ==
  note: VAS Actuation
  phiKnee : Inport
  StimVas : Inport  Port=2
  " VAS Golgi Tendon Organs" : Gain
  Gain : Gain  Gain=-1
  Mux9 : Mux  Inputs=5
  Product4 : Product  RndMeth=Zero
  Terminator9 : Terminator
  VAS : Subsystem
  VAS Link : Subsystem
  VAS loop delay : TransportDelay  DelayTime=MidDelay
  TauVas : Outport
  FmVas : Outport  Port=2
  wires:
  VAS Link/1(lmtu [m]) -> VAS/2(lmtc [m])
  Product4/1 -> Gain/1
  VAS/5(A) -> Mux9/5
  VAS/1(Fmtc) -> Product4/2, " VAS Golgi Tendon Organs"/1, Mux9/1
  VAS Link/2(lever [m]) -> Product4/1
  Mux9/1 -> Terminator9/1
  VAS/4(Lse) -> Mux9/4
  VAS/3(Vce) -> Mux9/3
  VAS/2(Lce) -> Mux9/2
  phiKnee/1 -> VAS Link/1(phi23 [rad])
  StimVas/1 -> VAS/1(STIM)
  Gain/1 -> TauVas/1
  " VAS Golgi Tendon Organs"/1 -> VAS loop delay/1
  VAS loop delay/1 -> FmVas/1

== system nmc/Full Body Control/Left Side/AnkleJoint left ==
  note: Ankle Joint
  phidphiAnkle : Inport
  PreTauAnkle : Inport  Port=2
  " Ankle Joint Limits" : Subsystem
  Demux : Demux  Outputs=2
  Sum : Sum  Inputs=|++
  Sum of Elements : Sum  Inputs=+
  TauAnkle : Outport
  wires:
  Sum of Elements/1 -> Sum/2
  Sum/1 -> TauAnkle/1
  " Ankle Joint Limits"/1(M_stop [Nm]) -> Sum/1
  phidphiAnkle/1 -> Demux/1
  PreTauAnkle/1 -> Sum of Elements/1
  Demux/2 -> " Ankle Joint Limits"/2(dphi [rad/s])
  Demux/1 -> " Ankle Joint Limits"/1(phi [rad])

== system nmc/Full Body Control/Left Side/HipJoint left ==
  note: Hip Joint
  phidphiHip : Inport
  PreTauHip : Inport  Port=2
  Demux2 : Demux  Outputs=2
  Hip Joint Limits : Subsystem
  Sum of Elements : Sum  Inputs=+
  Sum16 : Sum  Inputs=|++
  TauHip : Outport
  wires:
  Sum of Elements/1 -> Sum16/2
  PreTauHip/1 -> Sum of Elements/1
  Sum16/1 -> TauHip/1
  Hip Joint Limits/1(M_stop [Nm]) -> Sum16/1
  Demux2/2 -> Hip Joint Limits/2(dphi [rad/s])
  Demux2/1 -> Hip Joint Limits/1(phi [rad])
  phidphiHip/1 -> Demux2/1

== system nmc/Full Body Control/Left Side/KneeJoint left ==
  note: Knee Joint
  phidphiKnee : Inport
  PreTauKnee : Inport  Port=2
  Demux1 : Demux  Outputs=2
  Gain : Gain  Gain=-1
  Knee Joint Limits : Subsystem
  Sum : Sum  Inputs=|++
  Sum of Elements : Sum  Inputs=+
  TauKnee : Outport
  wires:
  Gain/1 -> Sum/2
  Sum of Elements/1 -> Gain/1
  PreTauKnee/1 -> Sum of Elements/1
  Sum/1 -> TauKnee/1
  Knee Joint Limits/1(M_stop [Nm]) -> Sum/1
  phidphiKnee/1 -> Demux1/1
  Demux1/2 -> Knee Joint Limits/2(dphi [rad/s])
  Demux1/1 -> Knee Joint Limits/1(phi [rad])

== system nmc/LeftSwing/GenerateAndSaveNominalShape/SaveToWorkspace ==
  In1 : Inport
  Enable : EnablePort
  saveGto : ToWorkspace  VariableName=NominalShape1  SaveFormat=Structure  SampleTime=-1
      settings: MaxDataPoints=1
  wires:
  In1/1 -> saveGto/1

== system nmc/Lopes/Left Side/HipJoint left ==
  note: Hip Joint
  phidphiHip : Inport
  PreTauHip : Inport  Port=2
  Demux2 : Demux  Outputs=2
  Hip Joint Limits : Subsystem
  Sum of Elements : Sum  Inputs=+
  Sum16 : Sum  Inputs=|++
  TauHip : Outport
  wires:
  Sum of Elements/1 -> Sum16/2
  PreTauHip/1 -> Sum of Elements/1
  Sum16/1 -> TauHip/1
  Hip Joint Limits/1(M_stop [Nm]) -> Sum16/1
  Demux2/2 -> Hip Joint Limits/2(dphi [rad/s])
  Demux2/1 -> Hip Joint Limits/1(phi [rad])
  phidphiHip/1 -> Demux2/1

== system nmc/Lopes/Left Side/KneeJoint left ==
  note: Knee Joint
  phidphiKnee : Inport
  PreTauKnee : Inport  Port=2
  Demux1 : Demux  Outputs=2
  Gain : Gain  Gain=-1
  Knee Joint Limits : Subsystem
  Sum : Sum  Inputs=|++
  Sum of Elements : Sum  Inputs=+
  TauKnee : Outport
  wires:
  Gain/1 -> Sum/2
  Sum of Elements/1 -> Gain/1
  PreTauKnee/1 -> Sum of Elements/1
  Sum/1 -> TauKnee/1
  Knee Joint Limits/1(M_stop [Nm]) -> Sum/1
  phidphiKnee/1 -> Demux1/1
  Demux1/2 -> Knee Joint Limits/2(dphi [rad/s])
  Demux1/1 -> Knee Joint Limits/1(phi [rad])

== system nmc/NMC Joints/AnkleJoint/ Ankle Joint Limits ==
  note: Ankle Joint Limits
  phi [rad] : Inport
  dphi [rad/s] : Inport  Port=2
  Gain1 : Gain  Gain=c_jointstop
  Gain2 : Gain  Gain=-1
  Gain3 : Gain  Gain=c_jointstop
  Gain4 : Gain  Gain=1/w_max_jointstop
  Limit Ankle Range : simulink/Logic and Bit Operations/Interval Test  IntervalClosedRight=on  uplimit=phi12_UpLimit + 40*pi/180  IntervalClosedLeft=on  lowlimit=phi12_LowLimit - 40*pi/180  OutDataTypeStr=boolean
  Logical Operator3 : Logic  Operator=NOT  AllPortsSameDT=off  OutDataTypeStr=boolean
  Mux1 : Mux  Inputs=2
  Mux3 : Mux  Inputs=2
  Overextension Torque : Fcn  Expr="- u(1)  *  (1-u(2)) * (u(2)<1) * (u(1)>0)"
  Overflexion Torque : Fcn  Expr="- u(1)  *  (1-u(2)) * (u(2)<1) * (u(1)<0)"
  Stop Simulation1 : Stop  Commented=on
  Sum : Sum  Inputs=|+-
  Sum1 : Sum  Inputs=|+-
  Sum2 : Sum
  overextension angle : Constant  Value=phi12_UpLimit
  overflexion angle : Constant  Value=phi12_LowLimit
  M_stop [Nm] : Outport
  wires:
  Mux3/1 -> Overextension Torque/1
  Gain3/1 -> Mux3/1
  dphi [rad/s]/1 -> Gain4/1
  overextension angle/1 -> Sum/2
  phi [rad]/1 -> Sum/1, Sum1/1, Limit Ankle Range/1
  Sum/1 -> Gain3/1
  Gain4/1 -> Gain2/1, Mux1/2
  Gain1/1 -> Mux1/1
  Sum1/1 -> Gain1/1
  overflexion angle/1 -> Sum1/2
  Mux1/1 -> Overflexion Torque/1
  Sum2/1 -> M_stop [Nm]/1
  Gain2/1 -> Mux3/2
  Overflexion Torque/1 -> Sum2/2
  Overextension Torque/1 -> Sum2/1
  Limit Ankle Range/1 -> Logical Operator3/1
  Logical Operator3/1 -> Stop Simulation1/1

== system nmc/NMC Joints/HipJoint/Hip Joint Limits ==
  note: Hip Joint Limits
  phi [rad] : Inport
  dphi [rad/s] : Inport  Port=2
  Gain2 : Gain  Gain=-1
  Gain3 : Gain  Gain=c_jointstop
  Gain4 : Gain  Gain=1/w_max_jointstop
  Limit Hip Range : simulink/Logic and Bit Operations/Interval Test  IntervalClosedRight=on  uplimit=phi34_UpLimit + 30*pi/180  IntervalClosedLeft=on  lowlimit=10*pi/180  OutDataTypeStr=boolean
  Logical Operator3 : Logic  Operator=NOT  AllPortsSameDT=off  OutDataTypeStr=boolean
  Mux3 : Mux  Inputs=2
  Overextension Torque : Fcn  Expr="- u(1)  *  (1-u(2)) * (u(2)<1) * (u(1)>0)"
  Stop Simulation1 : Stop  Commented=on
  Sum : Sum  Inputs=|+-
  overextension angle : Constant  Value=phi34_UpLimit
  M_stop [Nm] : Outport
  wires:
  Mux3/1 -> Overextension Torque/1
  Gain3/1 -> Mux3/1
  dphi [rad/s]/1 -> Gain4/1
  overextension angle/1 -> Sum/2
  phi [rad]/1 -> Sum/1, Limit Hip Range/1
  Sum/1 -> Gain3/1
  Gain4/1 -> Gain2/1
  Gain2/1 -> Mux3/2
  Overextension Torque/1 -> M_stop [Nm]/1
  Limit Hip Range/1 -> Logical Operator3/1
  Logical Operator3/1 -> Stop Simulation1/1

== system nmc/NMC Joints/KneeJoint/Knee Joint Limits ==
  note: Knee Joint Limits
  phi [rad] : Inport
  dphi [rad/s] : Inport  Port=2
  Gain2 : Gain  Gain=-1
  Gain3 : Gain  Gain=c_jointstop
  Gain4 : Gain  Gain=1/w_max_jointstop
  Limit Knee Range : simulink/Logic and Bit Operations/Interval Test  IntervalClosedRight=on  uplimit=185*pi/180  IntervalClosedLeft=on  lowlimit=40*pi/180  OutDataTypeStr=boolean
  Logical Operator3 : Logic  Operator=NOT  AllPortsSameDT=off  OutDataTypeStr=boolean
  Mux3 : Mux  Inputs=2
  Overextension Torque : Fcn  Expr="- u(1)  *  (1-u(2)) * (u(2)<1) * (u(1)>0)"
  Stop Simulation1 : Stop  Commented=on
  Sum : Sum  Inputs=|+-
  overextension angle : Constant  Value=phi23_UpLimit
  M_stop [Nm] : Outport
  wires:
  Mux3/1 -> Overextension Torque/1
  Gain3/1 -> Mux3/1
  dphi [rad/s]/1 -> Gain4/1
  overextension angle/1 -> Sum/2
  phi [rad]/1 -> Sum/1, Limit Knee Range/1
  Sum/1 -> Gain3/1
  Gain4/1 -> Gain2/1
  Gain2/1 -> Mux3/2
  Overextension Torque/1 -> M_stop [Nm]/1
  Limit Knee Range/1 -> Logical Operator3/1
  Logical Operator3/1 -> Stop Simulation1/1

== system nmc/NMC Muscles/GAS Muscle/GAS Actuation  ==
  note: GAS Actuation
  phiKnee : Inport
  phiAnkle : Inport  Port=2
  StimGas : Inport  Port=3
  " GAS" : Subsystem
  " GAS Golgi Tendon Organs" : Gain
  GAS Link : Subsystem
  GAS loop delay : TransportDelay  DelayTime=LongDelay
  Mux2 : Mux  Inputs=5
  Product2 : Product  RndMeth=Zero
  Product3 : Product  RndMeth=Zero
  Terminator2 : Terminator
  TauGasKnee : Outport
  TauGasAnkle : Outport  Port=2
  FmGas : Outport  Port=3
  tag scope: GASL_VM=global
  wires:
  GAS loop delay/1 -> FmGas/1
  " GAS Golgi Tendon Organs"/1 -> GAS loop delay/1
  Product2/1 -> TauGasAnkle/1
  StimGas/1 -> " GAS"/1(STIM)
  phiAnkle/1 -> GAS Link/2(phi12 [rad])
  phiKnee/1 -> GAS Link/1(phi23 [rad])
  " GAS"/2(Lce) -> Mux2/2
  " GAS"/3(Vce) -> Mux2/3
  " GAS"/4(Lse) -> Mux2/4
  Mux2/1 -> Terminator2/1, [GASL_VM]
  " GAS"/5(A) -> Mux2/5
  Product3/1 -> TauGasKnee/1
  GAS Link/1(lmtu [m]) -> " GAS"/2(lmtc [m])
  GAS Link/2(lever23 [m]) -> Product3/2
  GAS Link/3(lever12 [m]) -> Product2/2
  " GAS"/1(Fmtc) -> Mux2/1, " GAS Golgi Tendon Organs"/1, Product3/1, Product2/1

== system nmc/NMC Muscles/GAS Muscle/GAS Control ==
  note: GAS sControl
  FmGAS : Inport
  StanceSwing : Inport  Port=2
  " Swing Phase" : Subsystem  TreatAsAtomicUnit=on
  "ANMC STIM " : Concatenate  NumInputs=1
  Logical Operator : Logic  Operator=NOT  AllPortsSameDT=off  OutDataTypeStr=boolean
  Saturation17 : Saturate  UpperLimit=1  LowerLimit=0.01  ZeroCross=off
  Stance Phase : Subsystem  TreatAsAtomicUnit=on
  Sum18 : Sum
  StimGAS : Outport
  wires:
  "ANMC STIM "/1 -> StimGAS/1
  Stance Phase/1(StimGAS) -> Sum18/1
  Saturation17/1 -> "ANMC STIM "/1
  Sum18/1 -> Saturation17/1
  " Swing Phase"/1(StimGAS) -> Sum18/2
  StanceSwing/1 -> Stance Phase/Enable, Logical Operator/1
  FmGAS/1 -> Stance Phase/1(FmGAS)
  Logical Operator/1 -> " Swing Phase"/Enable

== system nmc/NMC Muscles/GLU Muscle/GLU Actuation ==
  note: GLU Actuation
  phiHip : Inport
  StimGlu : Inport  Port=2
  " GLU" : Subsystem
  " GLU Fm loop delay" : TransportDelay  DelayTime=ShortDelay
  GLU Golgi Tendon Organs : Gain
  GLU Link : Subsystem
  Mux : Mux  Inputs=5
  Product6 : Product  RndMeth=Zero
  Terminator : Terminator
  TauGlu : Outport
  FmGlu : Outport  Port=2
  tag scope: GLUR_VM=global
  wires:
  " GLU Fm loop delay"/1 -> FmGlu/1
  phiHip/1 -> GLU Link/1(phi34 [rad])
  Mux/1 -> Terminator/1, [GLUR_VM]
  " GLU"/4(Lse) -> Mux/4
  " GLU"/3(Vce) -> Mux/3
  " GLU"/2(Lce) -> Mux/2
  GLU Golgi Tendon Organs/1 -> " GLU Fm loop delay"/1
  " GLU"/5(A) -> Mux/5
  GLU Link/2(lever [m]) -> Product6/2
  GLU Link/1(lmtu [m]) -> " GLU"/2(lmtc [m])
  Product6/1 -> TauGlu/1
  StimGlu/1 -> " GLU"/1(STIM)
  " GLU"/1(Fmtc) -> Mux/1, GLU Golgi Tendon Organs/1, Product6/1

== system nmc/NMC Muscles/GLU Muscle/GLU Control ==
  note: GLU Control
  FmGlu : Inport
  Theta : Inport  Port=2
  dTheta : Inport  Port=3
  CLdxThigh : Inport  Port=4
  OLonCL : Inport  Port=5
  StanceSwing : Inport  Port=6
  " Swing Phase" : Subsystem  TreatAsAtomicUnit=on
  "ANMC STIM " : Concatenate  NumInputs=1
  Logical Operator : Logic  Operator=NOT  AllPortsSameDT=off  OutDataTypeStr=boolean
  Saturation17 : Saturate  UpperLimit=1  LowerLimit=0.01  ZeroCross=off
  Stance Phase : Subsystem  TreatAsAtomicUnit=on
  Sum18 : Sum
  StimGlu : Outport
  wires:
  "ANMC STIM "/1 -> StimGlu/1
  StanceSwing/1 -> Stance Phase/Enable, Logical Operator/1
  OLonCL/1 -> Stance Phase/4(OLonCL)
  CLdxThigh/1 -> Stance Phase/3(CLdxThigh [N])
  Stance Phase/1(StimGLU) -> Sum18/1
  Theta/1 -> Stance Phase/1(Theta)
  dTheta/1 -> Stance Phase/2(dTheta [rad/s])
  Saturation17/1 -> "ANMC STIM "/1
  Sum18/1 -> Saturation17/1
  FmGlu/1 -> " Swing Phase"/1(FmGLU)
  " Swing Phase"/1(StimGLU) -> Sum18/2
  Logical Operator/1 -> " Swing Phase"/Enable

== system nmc/NMC Muscles/HFL Muscle /HFL Actuation ==
  note: HFL Actuation
  phiHip : Inport
  StimHFL : Inport  Port=2
  " HFL" : Subsystem
  " HFL Muscle Spindles" : Gain  Gain=1/loptHFL
  " HFL Link" : Subsystem
  Gain : Gain  Gain=-1
  HFL Lce loop delay : TransportDelay  DelayTime=ShortDelay
  Mux10 : Mux  Inputs=5
  Product7 : Product  RndMeth=Zero
  Saturation5 : Saturate  UpperLimit=inf  LowerLimit=0  ZeroCross=off
  Stimulation Bias5 : Constant  Value=LceOffsetHFL
  Sum24 : Sum  Inputs=-+|  SaturateOnIntegerOverflow=on  InputSameDT=on  OutDataTypeStr=Inherit: Same as first input
  Terminator10 : Terminator
  TauHFL : Outport
  LceHFL : Outport  Port=2
  wires:
  HFL Lce loop delay/1 -> LceHFL/1
  Gain/1 -> TauHFL/1
  Product7/1 -> Gain/1
  StimHFL/1 -> " HFL"/1(STIM)
  phiHip/1 -> " HFL Link"/1(phi34 [rad])
  " HFL"/3(Vce) -> Mux10/3
  " HFL"/4(Lse) -> Mux10/4
  Mux10/1 -> Terminator10/1
  Saturation5/1 -> HFL Lce loop delay/1
  Sum24/1 -> Saturation5/1
  " HFL Muscle Spindles"/1 -> Sum24/2
  " HFL Link"/2(lever [m]) -> Product7/1
  " HFL"/5(A) -> Mux10/5
  " HFL Link"/1(lmtu [m]) -> " HFL"/2(lmtc [m])
  " HFL"/2(Lce) -> Mux10/2, " HFL Muscle Spindles"/1
  " HFL"/1(Fmtc) -> Mux10/1, Product7/2
  Stimulation Bias5/1 -> Sum24/1

== system nmc/NMC Muscles/HFL Muscle /HFL Control ==
  note: HFL Control
  LceHFL : Inport
  Theta : Inport  Port=2
  dTheta : Inport  Port=3
  CLdxThigh : Inport  Port=4
  OLonCL : Inport  Port=5
  StanceSwing : Inport  Port=6
  "ANMC STIM " : Concatenate  NumInputs=1
  Logical Operator : Logic  Operator=NOT  AllPortsSameDT=off  OutDataTypeStr=boolean
  Saturation17 : Saturate  UpperLimit=1  LowerLimit=0.01  ZeroCross=off
  Stance Phase : Subsystem  TreatAsAtomicUnit=on
  Sum18 : Sum
  Swing Phase : Subsystem  TreatAsAtomicUnit=on
  StimHFL : Outport
  wires:
  "ANMC STIM "/1 -> StimHFL/1
  Logical Operator/1 -> Swing Phase/Enable
  Theta/1 -> Stance Phase/1(Theta)
  dTheta/1 -> Stance Phase/2(dTheta [rad/s])
  Stance Phase/2(Delta_Theta) -> Swing Phase/1(Delta_Theta)
  CLdxThigh/1 -> Stance Phase/3(CLdxThigh [N])
  Stance Phase/1(StimHFL) -> Sum18/1
  LceHFL/1 -> Swing Phase/2(LceHFL)
  StanceSwing/1 -> Logical Operator/1, Stance Phase/Enable
  Sum18/1 -> Saturation17/1
  Swing Phase/1(StimHFL) -> Sum18/2
  OLonCL/1 -> Stance Phase/4(OLonCL)
  Saturation17/1 -> "ANMC STIM "/1

== system nmc/NMC Muscles/HFL&HAM Muscles/HAM Actuation  ==
  note: HAM Actuation
  phiHip : Inport
  phiKnee : Inport  Port=2
  StimHam : Inport  Port=3
  " HAM Muscle Spindles" : Gain  Gain=1/loptHAM
  " HAM Fm loop delay" : TransportDelay  DelayTime=ShortDelay
  " HAM Link" : Subsystem
  HAM : Subsystem
  HAM Golgi Tendon Organs : Gain
  HAM Lce loop delay : TransportDelay  DelayTime=ShortDelay
  Mux1 : Mux  Inputs=5
  Product8 : Product  RndMeth=Zero
  Product9 : Product  RndMeth=Zero
  Saturation7 : Saturate  UpperLimit=inf  LowerLimit=0  ZeroCross=off
  Stimulation Bias7 : Constant  Value=LceOffsetHAM
  Sum26 : Sum  Inputs=-+|  SaturateOnIntegerOverflow=on  InputSameDT=on  OutDataTypeStr=Inherit: Same as first input
  Terminator1 : Terminator
  TauHamHip : Outport
  TauHamKnee : Outport  Port=2
  LceHam : Outport  Port=3
  FmHam : Outport  Port=4
  tag scope: HAMR_VM=global
  wires:
  " HAM Fm loop delay"/1 -> FmHam/1
  HAM Lce loop delay/1 -> LceHam/1
  Saturation7/1 -> HAM Lce loop delay/1
  StimHam/1 -> HAM/1(STIM)
  Product9/1 -> TauHamKnee/1
  Stimulation Bias7/1 -> Sum26/1
  HAM/3(Vce) -> Mux1/3
  HAM/4(Lse) -> Mux1/4
  Mux1/1 -> Terminator1/1, [HAMR_VM]
  Sum26/1 -> Saturation7/1
  " HAM Muscle Spindles"/1 -> Sum26/2
  HAM Golgi Tendon Organs/1 -> " HAM Fm loop delay"/1
  Product8/1 -> TauHamHip/1
  HAM/5(A) -> Mux1/5
  phiHip/1 -> " HAM Link"/1(phi34 [rad])
  " HAM Link"/3(lever23 [m]) -> Product9/2
  " HAM Link"/2(lever34 [m]) -> Product8/2
  " HAM Link"/1(lmtu [m]) -> HAM/2(lmtc [m])
  HAM/2(Lce) -> Mux1/2, " HAM Muscle Spindles"/1
  HAM/1(Fmtc) -> Mux1/1, HAM Golgi Tendon Organs/1, Product8/1, Product9/1
  phiKnee/1 -> " HAM Link"/2(phi23 [rad])

== system nmc/NMC Muscles/HFL&HAM Muscles/HFL Actuation ==
  note: HFL Actuation
  phiHip : Inport
  StimHFL : Inport  Port=2
  " HFL" : Subsystem
  " HFL Muscle Spindles" : Gain  Gain=1/loptHFL
  " HFL Link" : Subsystem
  Gain : Gain  Gain=-1
  HFL Lce loop delay : TransportDelay  DelayTime=ShortDelay
  Mux10 : Mux  Inputs=5
  Product7 : Product  RndMeth=Zero
  Saturation5 : Saturate  UpperLimit=inf  LowerLimit=0  ZeroCross=off
  Stimulation Bias5 : Constant  Value=LceOffsetHFL
  Sum24 : Sum  Inputs=-+|  SaturateOnIntegerOverflow=on  InputSameDT=on  OutDataTypeStr=Inherit: Same as first input
  Terminator10 : Terminator
  TauHFL : Outport
  LceHFL : Outport  Port=2
  tag scope: HFLR_VM=global
  wires:
  HFL Lce loop delay/1 -> LceHFL/1
  Gain/1 -> TauHFL/1
  Product7/1 -> Gain/1
  StimHFL/1 -> " HFL"/1(STIM)
  phiHip/1 -> " HFL Link"/1(phi34 [rad])
  " HFL"/3(Vce) -> Mux10/3
  " HFL"/4(Lse) -> Mux10/4
  Mux10/1 -> Terminator10/1, [HFLR_VM]
  Saturation5/1 -> HFL Lce loop delay/1
  Sum24/1 -> Saturation5/1
  " HFL Muscle Spindles"/1 -> Sum24/2
  " HFL Link"/2(lever [m]) -> Product7/1
  " HFL"/5(A) -> Mux10/5
  " HFL Link"/1(lmtu [m]) -> " HFL"/2(lmtc [m])
  " HFL"/2(Lce) -> Mux10/2, " HFL Muscle Spindles"/1
  " HFL"/1(Fmtc) -> Mux10/1, Product7/2
  Stimulation Bias5/1 -> Sum24/1
